simulink model "ksrbl_4k4t_hdtrig"  (Simulink 6.2)
settings: Solver=ode45  StartTime=0.0  StopTime=20000  RelTol=1e-3
libraries: xbsIndex_r3 x1214, casper_library x120, xps_library x20
(part 12 of 26)

== system ksrbl_4k4t_hdtrig/pfb_fir_real/pol1_in2_first_tap/pfb_coeff_gen ==
  din : Inport  Port=1  LatchInput=off
  sync : Inport  Port=2  LatchInput=off
  Concat : xbsIndex_r3/Concat  num_inputs=4  explicit_period=off  period=1  dbl_ovrd=off
  Counter : xbsIndex_r3/Counter  cnt_type=Free Running  n_bits=10  bin_pt=0  arith_type=Unsigned  start_count=0  cnt_to=Inf  cnt_by_val=1  operation=Up  explicit_period=on  period=1  load_pin=off  rst=on  en=off  dbl_ovrd=off  show_param=off  use_rpm=on  gen_core=off
      settings: xl_area=[0, 0, 0, 0, 0, 0, 0]
  Delay : xbsIndex_r3/Delay  latency=bram_latency+1  reg_retiming=off  explicit_period=off  period=1  en=off  accept_only_valid=off  init_zero=on  dbl_ovrd=off  show_param=off
      settings: xl_area=[0, 0, 0, 0, 0, 0, 0]
  Delay1 : xbsIndex_r3/Delay  latency=5  reg_retiming=off  explicit_period=off  period=1  en=off  accept_only_valid=off  init_zero=on  dbl_ovrd=off  show_param=off
      settings: xl_area=[0, 0, 0, 0, 0, 0, 0]
  ROM1 : xbsIndex_r3/ROM  depth=1024  initVector=[-9.76682041096655e-006 -4.88583422828188e-005 -8.79896057392605e-005 -0.000127161889042145 -0.00016637647283676 -0.000205634640104953 -0.000244937676118224 -0.000284286868390688 -0.000323683506631797 -0.000363128882699047 -0.000402624290550542 -0.000442171026197326 -0.000481770387655752 -0.000521423674899556 -0.000561132189811922 -0.000600897236137418 -0.000640720119433707 -0.000680602147023241 -0.000720544627944829 -0.000760548872904983 -0.000800616194229252 -0.000840747905813429 -0.000880945323074528 -0.000921209762901825 -0.000961542543607595 -0.00100194498487787 -0.00104241840772305 -0.00108296413442834 -0.00112358348850416 -0.00116427779463642 -0.00120504837863661 -0.0012458965673919 -0.00128682368881508 -0.00132783107179433 -0.00136892004614302 -0.00141009194254927 -0.00145134809252546 -0.00149268982835772 -0.00153411848305515 -0.00157563539029908 -0.00161724188439217 -0.00165893930020741 -0.00170072897313705 -0.00174261223904142 -0.00178459043419762 -0.00182666489524821 -0.00186883695914968 -0.00191110796312089 -0.00195347924459153 -0.00199595214115024 -0.00203852799049285 -0.0020812081303705 -0.00212399389853753 -0.0021668866326995 -0.00220988767046099 -0.00225299834927326 -0.00229622000638206 -0.00233955397877506 -0.00238300160312942 -0.00242656421575926 -0.00247024315256288 -0.00251403974897009 -0.00255795533988945 -0.00260199125965526 -0.0026461488419747 -0.00269042941987476 -0.00273483432564911 -0.002779364890805 -0.0028240224460099 -0.00286880832103828 -0.0029137238447182 -0.00295877034487785 -0.00300394914829205 -0.00304926158062866 -0.00309470896639497 -0.00314029262888394 -0.00318601389012054 -0.00323187407080781 -0.00327787449027308 -0.00332401646641397 -0.00337030131564441 -0.00341673035284064 -0.00346330489128705 -0.00351002624262205 -0.00355689571678388 -0.00360391462195635 -0.00365108426451447 -0.00369840594897025 -0.00374588097791812 -0.00379351065198066 -0.00384129626975395 -0.00388923912775315 -0.00393734052035792 -0.00398560173975772 -0.00403402407589725 -0.00408260881642171 -0.00413135724662209 -0.00418027064938035 -0.00422935030511474 -0.00427859749172478 -0.00432801348453662 -0.00437759955624789 -0.00442735697687297 -0.00447728701368796 -0.00452739093117563 -0.00457766999097051 -0.0046281254518038 -0.00467875856944828 -0.00472957059666325 -0.00478056278313946 -0.00483173637544388 -0.00488309261696466 -0.00493463274785586 -0.00498635800498232 -0.00503826962186448 -0.00509036882862308 -0.00514265685192399 -0.00519513491492299 -0.00524780423721044 -0.00530066603475603 -0.00535372151985359 -0.00540697190106568 -0.00546041838316842 -0.0055140621670961 -0.00556790444988593 -0.00562194642462277 -0.00567618928038374 -0.00573063420218297 -0.00578528237091635 -0.00584013496330611 -0.00589519315184559 -0.00595045810474401 -0.00600593098587103 -0.00606161295470161 -0.00611750516626069 -0.00617360877106786 -0.00622992491508224 -0.00628645473964713 -0.00634319938143482 -0.00640015997239141 -0.00645733763968154 -0.00651473350563325 -0.00657234868768286 -0.0066301842983197 -0.00668824144503117 -0.00674652123024745 -0.00680502475128651 -0.00686375310029912 -0.00692270736421366 -0.00698188862468126 -0.00704129795802075 -0.00710093643516373 -0.00716080512159964 -0.00722090507732094 -0.00728123735676814 -0.00734180300877511 -0.00740260307651418 -0.00746363859744146 -0.00752491060324215 -0.00758642011977578 -0.00764816816702166 -0.00771015575902429 -0.00777238390383876 -0.00783485360347625 -0.00789756585384965 -0.00796052164471904 -0.00802372195963744 -0.00808716777589637 -0.00815086006447168 -0.00821479978996931 -0.00827898791057111 -0.00834342537798073 -0.00840811313736961 -0.00847305212732294 -0.00853824327978569 -0.00860368752000887 -0.0086693857664955 -0.00873533893094703 -0.00880154791820957 -0.00886801362622019 -0.00893473694595353 -0.00900171876136809 -0.00906895994935291 -0.00913646137967425 -0.00920422391492213 -0.00927224841045724 -0.00934053571435778 -0.00940908666736627 -0.00947790210283668 ...(+16641 chars)]  arith_type="Signed  (2's comp)"  n_bits=8  bin_pt=7  latency=4  init_zero=on  explicit_period=off  period=1  rst=off  init_reg=0  en=off  dbl_ovrd=off  show_param=on  distributed_mem=off  use_rpm=on  gen_core=off
      settings: xl_area=[0, 0, 0, 0, 0, 0, 0]
  ROM2 : xbsIndex_r3/ROM  depth=1024  initVector=[0.000131921970750505 0.000661115706329907 0.00119272035746402 0.0017267379729317 0.00226317057708744 0.00280202016979086 0.0033432887263357 0.00388697819737954 0.00443309050887336 0.00498162756199214 0.00553259123306506 0.00608598337350598 0.00664180580974492 0.007200060343159 0.00776074875000423 0.00832387278134701 0.00888943416299681 0.00945743459543828 0.0100278757537642 0.0106007592876082 0.0111760868210785 0.0117538599526915 0.0123340802553053 0.0129167492760546 0.0135018685362848 0.014089439531487 0.0146794637312331 0.0152719425791115 0.0158668774926625 0.0164642698633149 0.0170641210563218 0.017666432410698 0.0182712052391564 0.0188784408280456 0.0194881404372878 0.0201003053003165 0.020714936624015 0.0213320355886546 0.0219516033478342 0.022573641028419 0.0231981497304806 0.0238251305272363 0.0244545844649899 0.0250865125630724 0.0257209158137819 0.0263577951823261 0.0269971516067631 0.0276389859979437 0.0282832992394532 0.0289300921875543 0.0295793656711302 0.0302311204916274 0.0308853574229995 0.0315420772116512 0.0322012805763827 0.0328629682083337 0.0335271407709293 0.0341937988998245 0.0348629432028505 0.03553457425996 0.0362086926231742 0.0368852988165293 0.0375643933360236 0.0382459766495644 0.0389300491969168 0.0396166113896508 0.0403056636110905 0.0409972062162624 0.0416912395318451 0.0423877638561186 0.0430867794589141 0.0437882865815643 0.0444922854368548 0.0451987762089736 0.0459077590534639 0.0466192340971753 0.0473332014382158 0.0480496611459042 0.0487686132607235 0.0494900577942736 0.0502139947292251 0.050940424019273 0.0516693455890916 0.0524007593342889 0.0531346651213613 0.0538710627876498 0.0546099521412954 0.0553513329611956 0.0560952049969606 0.0568415679688707 0.0575904215678336 0.0583417654553421 0.0590955992634319 0.0598519225946409 0.0606107350219676 0.0613720360888303 0.0621358253090273 0.0629021021666965 0.0636708661162761 0.0644421165824655 0.0652158529601864 0.0659920746145448 0.0667707808807927 0.0675519710642904 0.06833564444047 0.0691218002547983 0.06991043772274 0.0707015560297224 0.0714951543310997 0.0722912317521176 0.0730897873878786 0.0738908203033078 0.0746943295331192 0.0755003140817814 0.0763087729234851 0.0771197050021103 0.0779331092311937 0.0787489844938971 0.0795673296429756 0.0803881435007469 0.0812114248590605 0.0820371724792668 0.0828653850921882 0.0836960613980893 0.0845292000666476 0.0853647997369252 0.0862028590173405 0.0870433764856407 0.0878863506888735 0.0887317801433617 0.0895796633346752 0.0904299987176061 0.0912827847161418 0.0921380197234409 0.0929957021018077 0.0938558301826681 0.0947184022665451 0.0955834166230361 0.096450871490789 0.0973207650774799 0.0981930955597905 0.0990678610833867 0.0999450597628969 0.100824689681891 0.101706748892859 0.102591235417194 0.103478147245168 0.104367482335915 0.105259238617414 0.106153413986466 0.107050006308681 0.107949013418457 0.108850433118963 0.109754263182125 0.110660501348608 0.1115691453278 0.112480192797796 0.113393641405385 0.114309488766036 0.115227732463879 0.116148370051699 0.117071399050915 0.117996816951575 0.118924621212337 0.119854809260461 0.120787378491797 0.121722326270772 0.122659649930383 0.123599346772185 0.124541414066281 0.125485849051313 0.126432648934455 0.127381810891403 0.128333332066366 0.129287209572061 0.130243440489708 0.131202021869017 0.132162950728188 0.133126224053902 0.134091838801319 0.135059791894069 0.136030080224252 0.137002700652432 0.137977650007634 0.138954925087342 0.139934522657494 0.140916439452484 0.141900672175158 0.142887217496813 0.143876072057195 0.144867232464505 0.14586069529539 0.146856457094953 0.147854514376746 0.14885486362278 0.149857501283519 0.150862423777888 0.151869627493274 0.152879108785532 0.153890863978983 0.154904889366426 0.155921181209138 0.156939735736879 0.157960549147901 0.158983617608954 0.160008937255289 0.161036504190669 0.162066314487373 0.163098364186211 0.164132649296523 0.165169165796195 0.166207909631668 0.167248876717944 0.168292062938599 ...(+14481 chars)]  arith_type="Signed  (2's comp)"  n_bits=8  bin_pt=7  latency=4  init_zero=on  explicit_period=off  period=1  rst=off  init_reg=0  en=off  dbl_ovrd=off  show_param=on  distributed_mem=off  use_rpm=on  gen_core=off
      settings: xl_area=[0, 0, 0, 0, 0, 0, 0]
  ROM3 : xbsIndex_r3/ROM  depth=1024  initVector=[0.999999825837027 0.999996525507456 0.999989005195528 0.999977264973965 0.99996130495613 0.999941125296029 0.999916726188311 0.999888107868258 0.999855270611789 0.999818214735455 0.999776940596432 0.999731448592517 0.999681739162128 0.999627812784289 0.999569669978633 0.999507311305389 0.999440737365378 0.9993699488 0.999294946291236 0.999215730561625 0.999132302374269 0.999044662532811 0.998952811881432 0.998856751304836 0.99875648172824 0.998652004117363 0.99854331947841 0.998430428858063 0.998313333343463 0.998192034062199 0.998066532182293 0.997936828912181 0.997802925500702 0.99766482323708 0.997522523450905 0.997376027512119 0.997225336830994 0.997070452858119 0.996911377084375 0.996748111040919 0.996580656299165 0.996409014470759 0.996233187207562 0.996053176201627 0.995868983185177 0.99568060993058 0.99548805825033 0.99529132999702 0.99509042706332 0.994885351381949 0.994676104925654 0.99446268970718 0.994245107779247 0.99402336123452 0.993797452205585 0.993567382864918 0.993333155424858 0.993094772137579 0.992852235295059 0.992605547229049 0.992354710311045 0.992099726952256 0.991840599603573 0.991577330755534 0.991309922938296 0.991038378721597 0.990762700714727 0.990482891566491 0.990198953965174 0.989910890638509 0.989618704353637 0.989322397917074 0.989021974174674 0.988717436011588 0.988408786352235 0.988096028160251 0.987779164438462 0.987458198228839 0.987133132612458 0.986803970709462 0.986470715679019 0.986133370719281 0.98579193906734 0.98544642399919 0.985096828829681 0.984743156912476 0.984385411640009 0.984023596443436 0.983657714792597 0.983287770195967 0.982913766200606 0.982535706392122 0.982153594394616 0.981767433870638 0.98137722852114 0.980982982085426 0.980584698341101 0.980182381104029 0.979776034228275 0.979365661606058 0.978951267167703 0.978532854881583 0.978110428754075 0.9776839928295 0.977253551190078 0.976819107955867 0.976380667284716 0.975938233372204 0.975491810451593 0.975041402793765 0.974587014707173 0.974128650537779 0.973666314669001 0.973200011521655 0.972729745553898 0.972255521261167 0.971777343176124 0.971295215868593 0.970809143945505 0.970319132050834 0.96982518486554 0.969327307107503 0.968825503531467 0.968319778928974 0.967810138128303 0.967296585994409 0.966779127428855 0.966257767369753 0.965732510791697 0.965203362705698 0.964670328159119 0.964133412235612 0.963592620055047 0.963047956773451 0.962499427582933 0.961947037711624 0.961390792423608 0.960830697018847 0.96026675683312 0.959698977237948 0.959127363640528 0.958551921483659 0.957972656245676 0.957389573440371 0.956802678616931 0.956211977359858 0.955617475288901 0.955019178058979 0.954417091360111 0.953811220917342 0.953201572490665 0.95258815187495 0.951970964899866 0.951350017429808 0.950725315363818 0.95009686463551 0.949464671212993 0.948828741098791 0.948189080329771 0.947545694977056 0.946898591145955 0.946247774975876 0.945593252640254 0.944935030346464 0.944273114335743 0.943607510883112 0.942938226297289 0.942265266920612 0.941588639128955 0.940908349331643 0.940224403971374 0.939536809524131 0.9388455724991 0.938150699438584 0.937452196917922 0.936750071545399 0.936044329962165 0.935334978842145 0.934622024891954 0.933905474850811 0.933185335490453 0.932461613615042 0.931734316061084 0.931003449697333 0.930269021424711 0.92953103817621 0.928789506916806 0.928044434643373 0.927295828384584 0.926543695200827 0.925788042184112 0.925028876457976 0.924266205177398 0.923500035528698 0.922730374729451 0.92195723002839 0.921180608705314 0.920400518070993 0.919616965467075 0.91882995826599 0.918039503870855 0.917245609715377 0.916448283263764 0.915647532010617 0.914843363480844 0.914035785229557 0.913224804841978 0.912410429933337 0.911592668148778 0.910771527163259 0.909947014681451 0.909119138437644 0.908287906195642 0.907453325748664 0.906615404919247 0.905774151559141 0.904929573549212 0.904081678799337 0.903230475248304 0.90237597086371 0.901518173641857 0.900657091607652 0.899792732814501 ...(+14492 chars)]  arith_type="Signed  (2's comp)"  n_bits=8  bin_pt=7  latency=4  init_zero=on  explicit_period=off  period=1  rst=off  init_reg=0  en=off  dbl_ovrd=off  show_param=off  distributed_mem=off  use_rpm=on  gen_core=off
      settings: xl_area=[0, 0, 0, 0, 0, 0, 0]
  ROM4 : xbsIndex_r3/ROM  depth=1024  initVector=[-0.000131728390195665 -0.000657137616413107 -0.00118014149426112 -0.00170074215927932 -0.00221894177110112 -0.00273474251338165 -0.0032481465937247 -0.00375915624360981 -0.00426777371831864 -0.00477400129686187 -0.00527784128190513 -0.00577929599969462 -0.00627836779998326 -0.00677505905595573 -0.00726937216415374 -0.0077613095444006 -0.00825087363972626 -0.00873806691629138 -0.00922289186331156 -0.00970535099298095 -0.0101854468403962 -0.0106631819634797 -0.0111385589429024 -0.011611580382007 -0.0120822489067307 -0.0125505671655272 -0.0130165378292889 -0.013480163591269 -0.0139414471670031 -0.0144003912942307 -0.0148569987328161 -0.0153112722646696 -0.0157632146936685 -0.0162128288455767 -0.0166601175679663 -0.0171050837301363 -0.0175477302230336 -0.0179880599591717 -0.0184260758725504 -0.0188617809185754 -0.0192951780739766 -0.019726270336727 -0.0201550607259614 -0.0205815522818946 -0.0210057480657395 -0.0214276511596248 -0.021847264666513 -0.0222645917101176 -0.0226796354348205 -0.0230923990055887 -0.0235028856078918 -0.0239110984476181 -0.0243170407509911 -0.024720715764486 -0.0251221267547457 -0.0255212770084962 -0.025918169832463 -0.026312808553286 -0.0267051965174352 -0.0270953370911251 -0.0274832336602305 -0.0278688896302007 -0.0282523084259741 -0.0286334934918925 -0.0290124482916153 -0.0293891763080338 -0.0297636810431845 -0.0301359660181631 -0.0305060347730379 -0.0308738908667631 -0.0312395378770917 -0.0316029794004887 -0.0319642190520439 -0.0323232604653844 -0.032680107292587 -0.0330347632040907 -0.0333872318886087 -0.0337375170530403 -0.0340856224223828 -0.0344315517396432 -0.0347753087657498 -0.035116897279463 -0.0354563210772873 -0.0357935839733817 -0.0361286897994709 -0.036461642404756 -0.0367924456558251 -0.0371211034365639 -0.0374476196480654 -0.0377719982085411 -0.0380942430532303 -0.0384143581343102 -0.0387323474208055 -0.0390482148984986 -0.0393619645698384 -0.0396736004538501 -0.0399831265860443 -0.0402905470183263 -0.0405958658189047 -0.0408990870722006 -0.0412002148787565 -0.0414992533551443 -0.0417962066338746 -0.0420910788633042 -0.0423838742075453 -0.0426745968463732 -0.0429632509751339 -0.0432498408046531 -0.043534370561143 -0.0438168444861108 -0.0440972668362657 -0.0443756418834268 -0.0446519739144304 -0.0449262672310373 -0.04519852614984 -0.0454687550021697 -0.0457369581340039 -0.0460031399058722 -0.0462673046927643 -0.046529456884036 -0.0467896008833162 -0.0470477411084133 -0.0473038819912217 -0.0475580279776282 -0.0478101835274186 -0.048060353114183 -0.0483085412252234 -0.0485547523614585 -0.0487989910373301 -0.0490412617807094 -0.0492815691328025 -0.0495199176480561 -0.0497563118940633 -0.0499907564514693 -0.0502232559138771 -0.0504538148877529 -0.0506824379923311 -0.0509091298595204 -0.051133895133809 -0.0513567384721693 -0.0515776645439637 -0.0517966780308497 -0.0520137836266847 -0.0522289860374311 -0.0524422899810619 -0.0526537001874647 -0.0528632213983475 -0.0530708583671429 -0.0532766158589133 -0.0534804986502556 -0.053682511529206 -0.0538826592951445 -0.0540809467586999 -0.0542773787416539 -0.0544719600768464 -0.0546646956080796 -0.0548555901900226 -0.0550446486881159 -0.0552318759784763 -0.0554172769478006 -0.0556008564932707 -0.0557826195224576 -0.0559625709532263 -0.0561407157136394 -0.0563170587418624 -0.0564916049860671 -0.0566643594043367 -0.0568353269645696 -0.0570045126443842 -0.0571719214310226 -0.0573375583212555 -0.0575014283212861 -0.0576635364466545 -0.057823887722142 -0.0579824871816754 -0.0581393398682313 -0.0582944508337403 -0.0584478251389912 -0.0585994678535357 -0.0587493840555924 -0.0588975788319511 -0.0590440572778771 -0.059188824497016 -0.0593318856012971 -0.059473245710839 -0.059612909953853 -0.0597508834665479 -0.0598871713930344 -0.0600217788852296 -0.0601547111027613 -0.0602859732128728 -0.0604155703903269 -0.0605435078173111 -0.0606697906833418 -0.0607944241851688 -0.0609174135266805 -0.0610387639188078 -0.0611584805794295 -0.0612765687332768 -0.0613930336118381 ...(+16616 chars)]  arith_type="Signed  (2's comp)"  n_bits=8  bin_pt=7  latency=4  init_zero=on  explicit_period=off  period=1  rst=off  init_reg=0  en=off  dbl_ovrd=off  show_param=off  distributed_mem=off  use_rpm=on  gen_core=off
      settings: xl_area=[0, 0, 0, 0, 0, 0, 0]
  Register : xbsIndex_r3/Register  init=0  reg_only_valid=off  explicit_period=off  period=1  rst=off  en=off  out_en=off  dbl_ovrd=off  show_param=off
      settings: xl_area=[0, 0, 0, 0, 0, 0, 0]
  Reinterpret{1..4} (4 alike) : xbsIndex_r3/Reinterpret  force_arith_type=on  arith_type=Unsigned  force_bin_pt=on  bin_pt=0  force_valid=on
  dout : Outport
  sync_out : Outport  Port=2
  coeff : Outport  Port=3
  wires:
  din/1 -> Delay1/1
  Delay1/1 -> dout/1
  sync/1 -> Counter/1, Delay/1
  Delay/1 -> sync_out/1
  Concat/1 -> Register/1
  Register/1 -> coeff/1
  Counter/1 -> ROM1/1, ROM2/1, ROM3/1, ROM4/1
  ROM1/1 -> Reinterpret1/1
  Reinterpret1/1 -> Concat/1
  ROM2/1 -> Reinterpret2/1
  Reinterpret2/1 -> Concat/2
  ROM3/1 -> Reinterpret3/1
  Reinterpret3/1 -> Concat/3
  ROM4/1 -> Reinterpret4/1
  Reinterpret4/1 -> Concat/4
